simulink model "control_model_new"  (R2018b)
settings: Solver=VariableStepAuto  StartTime=0.0  StopTime=40  RelTol=1e-3
libraries: simulink x2
settings Model: Creator=geraldlow  LastModifiedBy=geraldlow

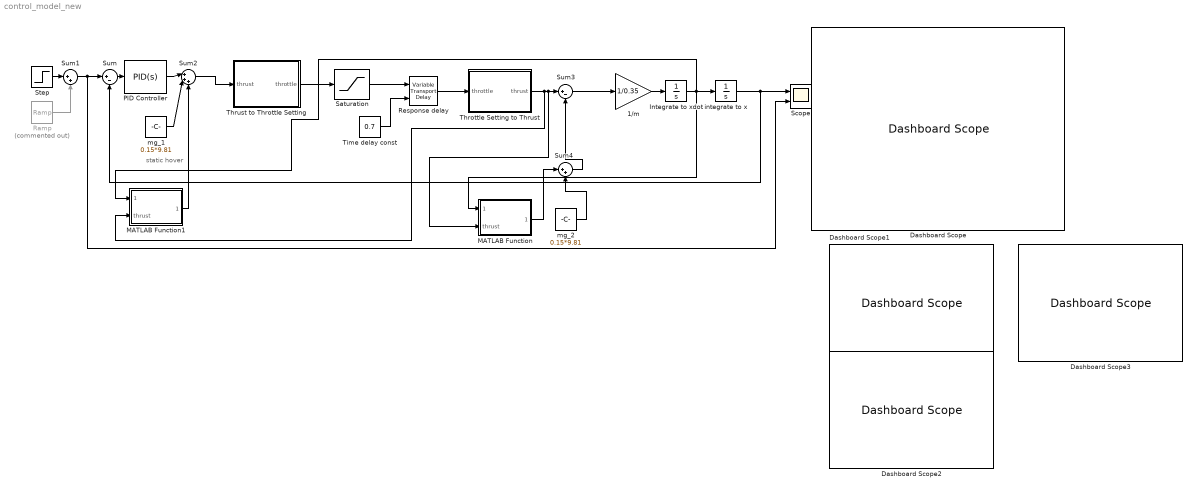
== system control_model_new ==
  note: static hover
  1/m : Gain  Gain=1/0.35
  Dashboard Scope : DashboardScope  WebBlockId=43
  Dashboard Scope1 : DashboardScope  WebBlockId=58
  Dashboard Scope2 : DashboardScope  WebBlockId=59
  Dashboard Scope3 : DashboardScope  WebBlockId=61
  Integrate to xdot : Integrator
  MATLAB Function : MATLAB Function  TreatAsAtomicUnit=on
  MATLAB Function1 : MATLAB Function  TreatAsAtomicUnit=on
  PID Controller : simulink/Continuous/PID Controller  Controller=PID  Form=Parallel  TimeDomain=Continuous-time  SampleTime=-1  IntegratorMethod=Forward Euler  FilterMethod=Forward Euler  ControllerParametersSource=internal  P=0.203  I=3.5e-03  D=0.45925  UseFilter=on  N=78.6717301092037  TunerSelectOption=Transfer Function Based (PID Tuner App)  InitialConditionSource=internal  InitialConditionForIntegrator=0  InitialConditionForFilter=0  DifferentiatorICPrevScaledInput=0  ExternalReset=none  TrackingMode=off  Kt=1  LimitOutput=off  UpperSaturationLimit=inf  LowerSaturationLimit=-inf  LinearizeAsGain=on  AntiWindupMode=none  Kb=1  POutMin=[]  POutMax=[]  IOutMin=[]  IOutMax=[]  DOutMin=[]  DOutMax=[]  NOutMin=[]  NOutMax=[]  SumOutMin=[]  SumOutMax=[]  SaturationOutMin=[]  SaturationOutMax=[]  PParamMin=[]  PParamMax=[]  IParamMin=[]  IParamMax=[]  DParamMin=[]  DParamMax=[]  NParamMin=[]  NParamMax=[]  KbParamMin=[]  KbParamMax=[]  KtParamMin=[]  KtParamMax=[]  KbOutMin=[]  KbOutMax=[]  KtOutMin=[]  KtOutMax=[]  IntegratorOutMin=[]  IntegratorOutMax=[]  FilterOutMin=[]  FilterOutMax=[]  SumI1OutMin=[]  SumI1OutMax=[]  SumI2OutMin=[]  SumI2OutMax=[]  SumI3OutMin=[]  SumI3OutMax=[]  SumI4OutMin=[]  SumI4OutMax=[]  SumDOutMin=[]  SumDOutMax=[]  DifferentiatorOutMin=[]  DifferentiatorOutMax=[]  FilterDiffOutCoefMin=[]  FilterDiffOutCoefMax=[]  ReciprocalOutMin=[]  ReciprocalOutMax=[]  SumDenOutMin=[]  SumDenOutMax=[]  SumNumOutMin=[]  SumNumOutMax=[]  DivideOutMin=[]  DivideOutMax=[]  IntegratorContinuousStateAttributes=''  IntegratorStateMustResolveToSignalObject=off  IntegratorRTWStateStorageClass=Auto  FilterContinuousStateAttributes=''  FilterStateMustResolveToSignalObject=off  FilterRTWStateStorageClass=Auto  ParallelPVariant=InternalParameters  IdealPVariant=Disabled  IVariant=InternalParameters  DVariant=InternalParameters  IntegratorVariant=Continuous  SatVariant=Disabled  AWVariant=Passthrough  PCopyVariant=Disabled  TRVariant=Disabled  FdbkBlocksVariant=Forward  IdealPFdbkVariant=Disabled  SatFdbkVariant=Disabled  DerivativeFilterVariant=ContFilter  NVariant=InternalParameters  NCopyVariant=Disabled  FilterICVariant=InternalICsFilter  IntegratorICVariant=InternalICs  ExternalResetVariant=Disabled  TRSumVariant=Passthrough  SumFdbkVariant=Disabled  SumVariant=Sum_PID
  Ramp : simulink/Sources/Ramp  Commented=on  slope=2  start=25  InitialOutput=0
  Response delay : VariableTransportDelay  MaximumDelay=10
  Saturation : Saturate  UpperLimit=100  LowerLimit=0
  Scope : Scope  NumInputPorts=2
  Step : Step  Time=2  After=10  SampleTime=0
  Sum : Sum  Inputs=|+-
  Sum1 : Sum  Inputs=|++
  Sum2 : Sum  Inputs=|+++
  Sum3 : Sum  Inputs=|+-
  Sum4 : Sum  Inputs=|++
  Throttle Setting to Thrust : MATLAB Function  TreatAsAtomicUnit=on
  Thrust to Throttle Setting : MATLAB Function  TreatAsAtomicUnit=on
  Time delay const : Constant  Value=0.7
  integrate to x : Integrator
  mg_1 : Constant  Value=0.15*9.81
  mg_2 : Constant  Value=0.15*9.81
  wires:
  Sum/1 -> PID Controller/1
  mg_1/1 -> Sum2/2
  Thrust to Throttle Setting/1(throttle) -> Saturation/1
  mg_2/1 -> Sum4/2
  1/m/1 -> Integrate to xdot/1
  Sum3/1 -> 1/m/1
  integrate to x/1 -> Scope/1, Sum/2
  PID Controller/1 -> Sum2/1
  Sum1/1 -> Scope/2, Sum/1
  Step/1 -> Sum1/1
  Ramp/1 -> Sum1/2
  Saturation/1 -> Response delay/1
  Response delay/1 -> Throttle Setting to Thrust/1(throttle)
  Time delay const/1 -> Response delay/2
  Sum2/1 -> Thrust to Throttle Setting/1(thrust)
  Sum4/1 -> Sum3/2
  MATLAB Function/1(friction) -> Sum4/1
  Throttle Setting to Thrust/1(thrust) -> MATLAB Function/2(thrust), Sum3/1, MATLAB Function1/2(thrust)
  Integrate to xdot/1 -> MATLAB Function1/1(velocity), MATLAB Function/1(velocity), integrate to x/1
  MATLAB Function1/1(friction) -> Sum2/3

== matlab function control_model_new/Throttle Setting to Thrust ==
  data: throttle input; thrust output
function thrust = fcn(throttle)
if throttle < 1
    thrust = 0;
elseif throttle > 88
    thrust=12.9492;
else
    thrust=0.981+(12.9492-0.981)/(88-1)*(throttle-1);
end
end

== matlab function control_model_new/Thrust to Throttle Setting ==
  data: thrust input; throttle output
function throttle = fcn(thrust)
throttle = (thrust / 0.0677)+1;
end

== matlab function control_model_new/MATLAB Function ==
  data: velocity input; friction output; thrust input
function friction   = fcn(velocity, thrust)
epsilon = 0.005; %small perturbation
mg = 0.15*9.81;
% Get reasonable values for x1, x2, l
x1 = 0.045;
x2 = 0.04;
l = 0.05;
netforce = thrust-mg; %mg should be a constant defined.
mu = 0.15; %coeff of dynamic friction
%static friction
if abs(velocity) < epsilon && abs(netforce) < 0.13*9.81 && netforce > 0
    friction = netforce;
elseif abs(velocity) < epsilon && abs(netforce) < 0.13*9.81 && netforce < 0
    friction = -netforce;
elseif velocity > 0
    friction=2*mu*(mg*x1-thrust*x2)/l;
elseif velocity < 0
    friction=-2*mu*(mg*x1-thrust*x2)/l;
else
    friction=0;
end

== matlab function control_model_new/MATLAB Function1 ==
  data: velocity input; friction output; thrust input
function friction   = fcn(velocity, thrust)
epsilon = 0.005; %small perturbation
mg = 0.15*9.81;
% Get reasonable values for x1, x2, l
x1 = 0.014;
x2 = x1/2;
l = 0.204;
netforce = thrust-mg; %mg should be a constant defined.
mu = 0.15; %coeff of dynamic friction
%static friction
if abs(velocity) < epsilon && abs(netforce) < 0.13*9.81 && netforce > 0
    friction = netforce;
elseif abs(velocity) < epsilon && abs(netforce) < 0.13*9.81 && netforce < 0
    friction = -netforce;
elseif velocity > 0
    friction=2*mu*(mg*x1-thrust*x2)/l;
elseif velocity < 0
    friction=-2*mu*(mg*x1-thrust*x2)/l;
else
    friction=0;
end
